simulink model "TCSmid"  (R2023a)
settings: Solver=VariableStepAuto  StartTime=0.0  StopTime=1000  RelTol=1e-3
libraries: slpidlib x1
settings Model: Creator=ibaad  LastModifiedBy=ibaad

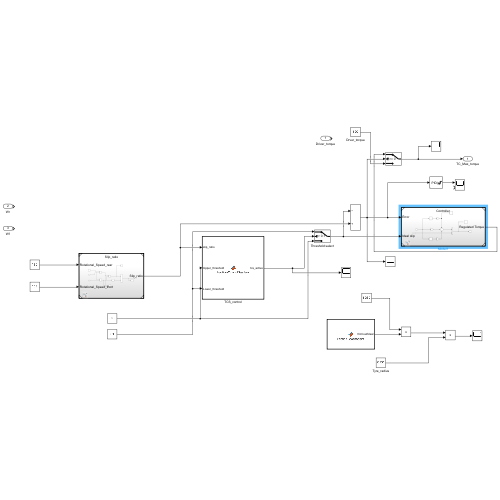
[thumbnail: Simulink's stored preview of the top-level diagram]
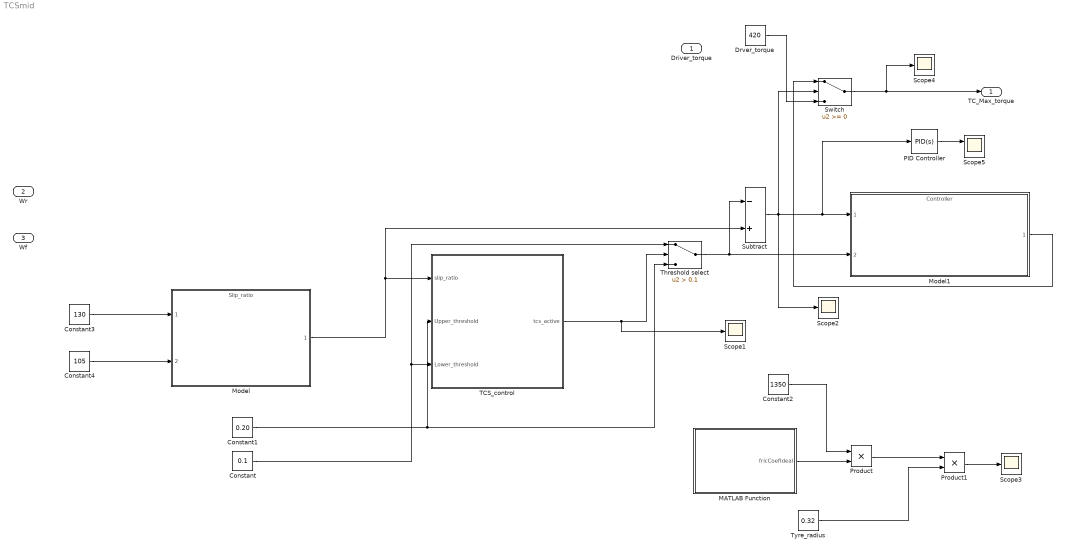
== system TCSmid ==
  Driver_torque : Inport
  Wr : Inport  Port=2
  Wf : Inport  Port=3
  Constant : Constant  Value=0.1
  Constant1 : Constant  Value=0.20
  Constant2 : Constant  Value=1350
  Constant3 : Constant  Value=130
  Constant4 : Constant  Value=105
  Drver_torque : Constant  Value=420
  MATLAB Function : MATLAB Function  TreatAsAtomicUnit=on
  Model : ModelReference  ModelNameDialog=Slip_ratio.slx  SimulationMode=Normal  ModelReferenceVersion=1.5
  Model1 : ModelReference  ModelNameDialog=Controller  SimulationMode=Normal  ModelReferenceVersion=1.6
  PID Controller : slpidlib/PID Controller  Controller=PID  Form=Parallel  TimeDomain=Continuous-time  UseExternalTs=off  SampleTime=-1  IntegratorMethod=Forward Euler  FilterMethod=Forward Euler  ControllerParametersSource=internal  P=45  I=15  UseKiTs=off  D=30  N=100  UseFilter=on  TunerSelectOption=Transfer Function Based (PID Tuner App)  InitialConditionSource=internal  InitialConditionForIntegrator=0  InitialConditionForFilter=0  DifferentiatorICPrevScaledInput=0  ExternalReset=none  TrackingMode=off  Kt=1  LimitOutput=on  SatLimitsSource=internal  UpperSaturationLimit=inf  LowerSaturationLimit=-inf  LinearizeAsGain=on  AntiWindupMode=clamping  Kb=1  LimitIntegrator=off  UpperIntegratorSaturationLimit=inf  LowerIntegratorSaturationLimit=-inf  POutMin=[]  POutMax=[]  IOutMin=[]  IOutMax=[]  DOutMin=[]  DOutMax=[]  NOutMin=[]  NOutMax=[]  SumOutMin=[]  SumOutMax=[]  SaturationOutMin=[]  SaturationOutMax=[]  PParamMin=[]  PParamMax=[]  IParamMin=[]  IParamMax=[]  DParamMin=[]  DParamMax=[]  NParamMin=[]  NParamMax=[]  KbParamMin=[]  KbParamMax=[]  KtParamMin=[]  KtParamMax=[]  KbOutMin=[]  KbOutMax=[]  KtOutMin=[]  KtOutMax=[]  IntegratorOutMin=[]  IntegratorOutMax=[]  FilterOutMin=[]  FilterOutMax=[]  SumI1OutMin=[]  SumI1OutMax=[]  SumI2OutMin=[]  SumI2OutMax=[]  SumI3OutMin=[]  SumI3OutMax=[]  SumI4OutMin=[]  SumI4OutMax=[]  SumDOutMin=[]  SumDOutMax=[]  DifferentiatorOutMin=[]  DifferentiatorOutMax=[]  FilterDiffOutCoefMin=[]  FilterDiffOutCoefMax=[]  ReciprocalOutMin=[]  ReciprocalOutMax=[]  SumDenOutMin=[]  SumDenOutMax=[]  SumNumOutMin=[]  SumNumOutMax=[]  DivideOutMin=[]  DivideOutMax=[]  UdiffTsProdOutMin=[]  UdiffTsProdOutMax=[]  NTsProdOutMin=[]  NTsProdOutMax=[]  UintegralTsProdOutMin=[]  UintegralTsProdOutMax=[]  UngainTsProdOutMin=[]  UngainTsProdOutMax=[]  ClampingZeroOutDataTypeStr=Inherit: Inherit via back propagation  ClampingZeroOutMin=[]  ClampingZeroOutMax=[]  FilterDenConstantOutDataTypeStr=Inherit: Inherit via back propagation  FilterDenConstantOutMin=[]  FilterDenConstantOutMax=[]  PCopyOutDataTypeStr=Inherit: Inherit via back propagation  PCopyOutMin=[]  PCopyOutMax=[]  NCopyOutDataTypeStr=Inherit: Inherit via back propagation  NCopyOutMin=[]  NCopyOutMax=[]  IntegratorContinuousStateAttributes=''  IntegratorStateMustResolveToSignalObject=off  IntegratorRTWStateStorageClass=Auto  FilterContinuousStateAttributes=''  FilterStateMustResolveToSignalObject=off  FilterRTWStateStorageClass=Auto  ParallelPVariant=InternalParameters  IdealPVariant=Disabled  IVariant=InternalParameters  DVariant=InternalParameters  IntegratorVariant=Continuous  SatVariant=Enabled  AWVariant=ContClampingParallel  PCopyVariant=Disabled  TRVariant=Disabled  FdbkBlocksVariant=Forward  IdealPFdbkVariant=Disabled  SatFdbkVariant=Disabled  DerivativeFilterVariant=ContFilter  NVariant=InternalParameters  NCopyVariant=Disabled  FilterICVariant=InternalICsFilter  IntegratorICVariant=InternalICs  ExternalResetVariant=Disabled  TRSumVariant=Passthrough  SumFdbkVariant=Disabled  SumVariant=Sum_PID  TsampFilterVariant=InternalTs  TsampNgainVariant=Passthrough  TsampIntegralVariant=Disabled_SignalSpec  ExternalSaturationOutDataTypeStr=Inherit: Same as second input
  Product : Product
  Product1 : Product
  Scope{1..4} (4 alike) : Scope
  Scope5 : Scope  NumInputPorts=2
  Subtract : Sum  Inputs=-+
  Switch : Switch  SaturateOnIntegerOverflow=off  InputSameDT=off
  TCS_control : MATLAB Function  TreatAsAtomicUnit=on
  Threshold select : Switch  Criteria=u2 > Threshold  Threshold=0.1  SaturateOnIntegerOverflow=off  InputSameDT=off
  Tyre_radius : Constant  Value=0.32
  TC_Max_torque : Outport
  wires:
  Model/1 -> Subtract/2, TCS_control/1(slip_ratio)
  Constant1/1 -> Threshold select/3, TCS_control/2(Upper_threshold)
  Constant/1 -> Threshold select/1, TCS_control/3(Lower_threshold)
  TCS_control/1(tcs_active) -> Scope1/1, Threshold select/2
  Threshold select/1 -> Model1/2, Subtract/1
  Subtract/1 -> PID Controller/1, Model1/1, Scope2/1, Switch/2
  Constant3/1 -> Model/1
  Constant4/1 -> Model/2
  Model1/1 -> Switch/1
  Switch/1 -> Scope4/1, TC_Max_torque/1
  MATLAB Function/1(fricCoefIdeal) -> Product/2
  Constant2/1 -> Product/1
  Product/1 -> Product1/1
  Tyre_radius/1 -> Product1/2
  Product1/1 -> Scope3/1
  Drver_torque/1 -> Switch/3
  PID Controller/1 -> Scope5/1

== matlab function TCSmid/MATLAB Function ==
  data: fricCoefIdeal output
function fricCoefIdeal = Friction_coefficient
    % TCS_ACTIVE Summary of this function goes here

    e = exp(1); % Mathematical constant e 
    % Friction curve as a function of slip ratio
    c1 = 1.2801; % Coef for dry asphalt
    c2 = 23.99; % Coef for dry asphalt
    c3 = 0.52; % Coef for dry asphalt

    slip_ratios = 0:0.05:0.4; % Create an array of slip ratios
    fricCoef = zeros(size(slip_ratios)); % Preallocate the array for efficiency

    for i = 1:length(slip_ratios)
        slip_ratio = slip_ratios(i);
        fricCoef(i) = c1 * (1 - e^(-c2 * slip_ratio)) - c3 * slip_ratio;
    end

 %   plot(slip_ratios, fricCoef); % Plot the entire array
   % xlabel("Slip Ratio");
%    ylabel("Longitudinal Friction Coefficient");
 %   title("Friction Coefficient vs. Slip Ratio Curve");
%    grid on;% Optionally, turn the grid on for better readability

    fricCoefIdeal = c1 * (1 - e^(-c2 * 0.19)) - c3 * 0.19;
end

== matlab function TCSmid/TCS_control ==
  settings: updateMethod=DISCRETE
  data: slip_ratio input; tcs_active output; Upper_threshold input; Lower_threshold input
function tcs_active  = tractionControlSystem(slip_ratio, Upper_threshold, Lower_threshold)

% For when TCS is inactive, motor outputs all the torque requested by the
% drive

persistent tcs_active_in;
if isempty(tcs_active_in)
    tcs_active_in = 0;
end

if slip_ratio > Upper_threshold
    tcs_active_in = 1;  
elseif slip_ratio < Lower_threshold
    tcs_active_in = 0;
end

tcs_active = tcs_active_in;

end
